simulink subsystem "SecondLink"  (R2023a)
settings: Solver=VariableStepAuto  StartTime=0.0  StopTime=10.0  RelTol=1e-3
undefined symbols (not defined in the file): K12
libraries: nesl_utility x4
settings Model: Creator=Alla  LastModifiedBy=Alla

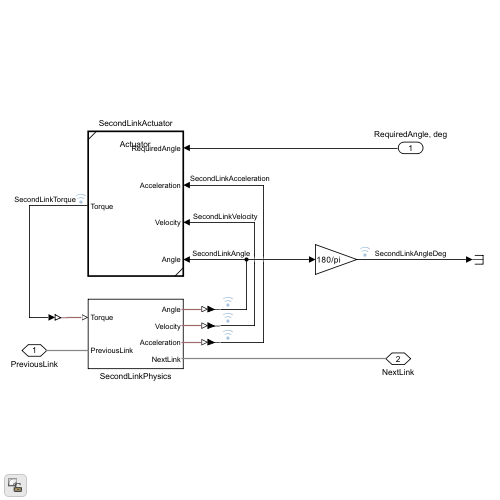
[thumbnail: Simulink's stored preview of the top-level diagram]
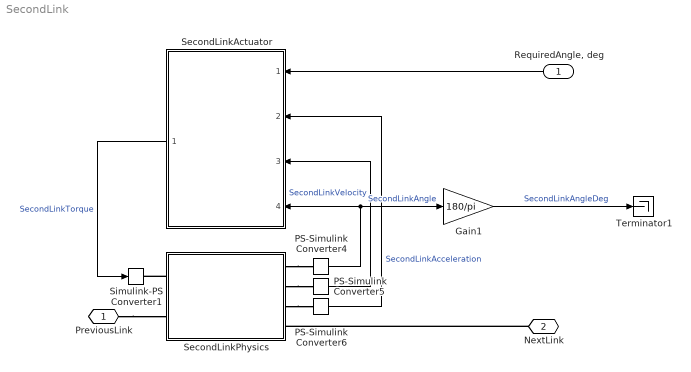
== system SecondLink ==
  "RequiredAngle, deg" : Inport
  Gain1 : Gain  Gain=180/pi
  PS-Simulink Converter4 : nesl_utility/PS-Simulink Converter  PhysicalDomain=network_engine_domain  SubClassName=ps_output  LeftPortType=input  RightPortType=output  PseudoPeriodic=off  Frequencies=[]  VectorFormat=inherit  Unit=inherit  AffineConversion=off
  PS-Simulink Converter5 : nesl_utility/PS-Simulink Converter  PhysicalDomain=network_engine_domain  SubClassName=ps_output  LeftPortType=input  RightPortType=output  PseudoPeriodic=off  Frequencies=[]  VectorFormat=inherit  Unit=inherit  AffineConversion=off
  PS-Simulink Converter6 : nesl_utility/PS-Simulink Converter  PhysicalDomain=network_engine_domain  SubClassName=ps_output  LeftPortType=input  RightPortType=output  PseudoPeriodic=off  Frequencies=[]  VectorFormat=inherit  Unit=inherit  AffineConversion=off
  SecondLinkActuator : Subsystem  TreatAsAtomicUnit=on  ReferencedSubsystem=Actuator  K=K12  Kv=K22  K1=K32  K2=K42  K3=K52
  SecondLinkPhysics : Subsystem  ReferencedSubsystem=SecondLinkPhysics
  Simulink-PS Converter1 : nesl_utility/Simulink-PS Converter  PhysicalDomain=network_engine_domain  SubClassName=ps_input  LeftPortType=input  RightPortType=output  PseudoPeriodic=off  Frequencies=[]  NoiseDistribution=none  NoiseParameters=[]  Unit=1  AffineConversion=off  FilteringAndDerivatives=provide  SimscapeFilterOrder=1  InputFilterTimeConstant=0.001  UdotUserProvided=0
  Terminator1 : Terminator
  PreviousLink : PMIOPort  Side=Left
  NextLink : PMIOPort  Port=2  Side=Right
  wires:
  SecondLinkActuator/1 -> Simulink-PS Converter1/1  "SecondLinkTorque"
  PS-Simulink Converter5/1 -> SecondLinkActuator/3  "SecondLinkVelocity"
  PS-Simulink Converter6/1 -> SecondLinkActuator/2  "SecondLinkAcceleration"
  "RequiredAngle, deg"/1 -> SecondLinkActuator/1
  Gain1/1 -> Terminator1/1  "SecondLinkAngleDeg"
  PS-Simulink Converter4/1 -> Gain1/1, SecondLinkActuator/4  "SecondLinkAngle"
  connections:
  SecondLinkPhysics/RConn1 -- PS-Simulink Converter4/LConn1
  SecondLinkPhysics/RConn2 -- PS-Simulink Converter5/LConn1
  SecondLinkPhysics/LConn1 -- Simulink-PS Converter1/RConn1
  SecondLinkPhysics/RConn3 -- PS-Simulink Converter6/LConn1
  NextLink/RConn1 -- SecondLinkPhysics/RConn4
  PreviousLink/RConn1 -- SecondLinkPhysics/LConn2
